simulink library "Byte_Multiplexers_Lib"  (R2023a)
settings: Solver=ode45  StartTime=0.0  StopTime=10.0  RelTol=1e-3  EnableMultiTasking=on
settings Model: Creator=uzivatel  LastModifiedBy=Jozko Mrkvicka
settings SolverCC: AlgebraicLoopSolver=TrustRegion
settings DataIOCC: LimitDataPoints=on  SaveFormat=Array  ReturnWorkspaceOutputs=off
settings OptimizationCC: LifeSpan=inf
settings DebuggingCC: UnderspecifiedInitializationDetection=Classic  MergeDetectMultiDrivingBlocksExec=none  SolverPrmCheckMsg=warning  UnconnectedInputMsg=warning  UnconnectedOutputMsg=warning  UnconnectedLineMsg=warning  StateNameClashWarn=warning  SFUnexpectedBacktrackingDiag=warning  SFNoUnconditionalDefaultTransitionDiag=warning  ArithmeticOperatorsInVariantConditions=warning
settings HardwareCC: ProdBitPerPointer=32  ProdBitPerSizeT=32  ProdBitPerPtrDiffT=32  ProdLargestAtomicFloat=None  ProdIntDivRoundTo=Undefined  ProdEndianess=Unspecified  ProdWordSize=32  ProdHWDeviceType=32-bit Generic
settings ModelReferenceCC: EnableRefExpFcnMdlSchedulingChecks=on  PropagateSignalLabelsOutOfModel=off
settings SFSimCC: SimUseLocalCustomCode=off  CustomCodeUndefinedFunction=UseInterfaceOnly
settings RTWCC: RTWUseLocalCustomCode=off
settings CodeAppCC: StateflowObjectComments=on
settings GRTTargetCC: TargetLangStandard=C89/C90 (ANSI)
settings ConfigComp: CovMetricSettings=dw  CovSaveCumulativeToWorkspaceVar=on  CovSaveSingleToWorkspaceVar=on  CovExternalEMLEnable=off

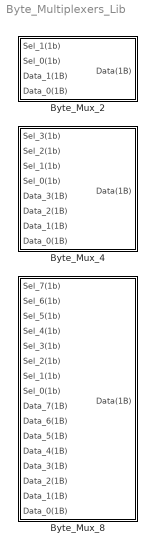
== system Byte_Multiplexers_Lib ==
  Byte_Mux_2 : Subsystem
  Byte_Mux_4 : Subsystem
  Byte_Mux_8 : Subsystem

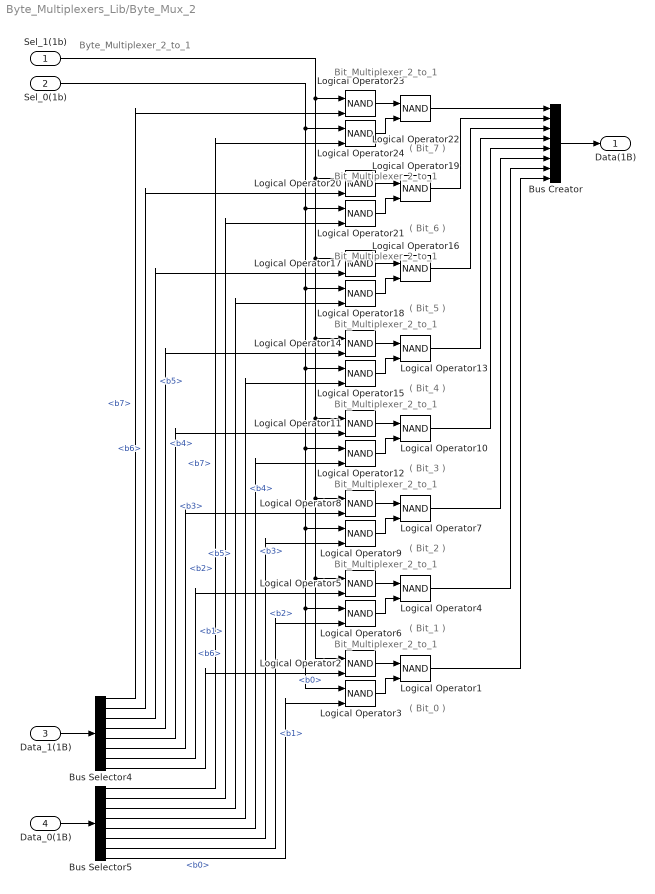
== system Byte_Multiplexers_Lib/Byte_Mux_2 ==
  note: ( Bit_0 )
  note: Bit_Multiplexer_2_to_1
  note: ( Bit_1 )
  note: Bit_Multiplexer_2_to_1
  note: ( Bit_2 )
  note: Bit_Multiplexer_2_to_1
  note: ( Bit_3 )
  note: Bit_Multiplexer_2_to_1
  note: ( Bit_4 )
  note: Bit_Multiplexer_2_to_1
  note: ( Bit_5 )
  note: Bit_Multiplexer_2_to_1
  note: ( Bit_6 )
  note: Bit_Multiplexer_2_to_1
  note: ( Bit_7 )
  note: Bit_Multiplexer_2_to_1
  note: Byte_Multiplexer_2_to_1
  Sel_1(1b) : Inport
  Sel_0(1b) : Inport  Port=2
  Data_1(1B) : Inport  Port=3
  Data_0(1B) : Inport  Port=4
  Bus Creator : BusCreator  Inputs=8
  Bus Selector4 : BusSelector  OutputSignals=b7,b6,b5,b4,b3,b2,b1,b0
  Bus Selector5 : BusSelector  OutputSignals=b7,b6,b5,b4,b3,b2,b1,b0
  Logical Operator{1..24} (24 alike) : Logic  Operator=NAND  IconShape=distinctive  AllPortsSameDT=off  OutDataTypeStr=boolean
  Data(1B) : Outport
  wires:
  Bus Creator/1 -> Data(1B)/1
  Bus Selector5/8 -> Logical Operator3/2  "<b0>"
  Bus Selector4/8 -> Logical Operator2/2  "<b0>"
  Bus Selector5/7 -> Logical Operator6/2  "<b1>"
  Bus Selector4/7 -> Logical Operator5/2  "<b1>"
  Bus Selector5/6 -> Logical Operator9/2  "<b2>"
  Bus Selector4/6 -> Logical Operator8/2  "<b2>"
  Bus Selector5/5 -> Logical Operator12/2  "<b3>"
  Bus Selector4/5 -> Logical Operator11/2  "<b3>"
  Bus Selector5/4 -> Logical Operator15/2  "<b4>"
  Bus Selector4/4 -> Logical Operator14/2  "<b4>"
  Bus Selector5/3 -> Logical Operator18/2  "<b5>"
  Bus Selector4/3 -> Logical Operator17/2  "<b5>"
  Bus Selector5/2 -> Logical Operator21/2  "<b6>"
  Bus Selector4/2 -> Logical Operator20/2  "<b6>"
  Bus Selector5/1 -> Logical Operator24/2  "<b7>"
  Bus Selector4/1 -> Logical Operator23/2  "<b7>"
  Sel_0(1b)/1 -> Logical Operator24/1, Logical Operator21/1, Logical Operator18/1, Logical Operator15/1, Logical Operator12/1, Logical Operator9/1, Logical Operator3/1, Logical Operator6/1
  Logical Operator19/1 -> Bus Creator/2
  Logical Operator13/1 -> Bus Creator/4
  Logical Operator7/1 -> Bus Creator/6
  Logical Operator1/1 -> Bus Creator/8
  Logical Operator4/1 -> Bus Creator/7
  Logical Operator10/1 -> Bus Creator/5
  Logical Operator16/1 -> Bus Creator/3
  Logical Operator22/1 -> Bus Creator/1
  Data_0(1B)/1 -> Bus Selector5/1
  Data_1(1B)/1 -> Bus Selector4/1
  Logical Operator3/1 -> Logical Operator1/2
  Logical Operator2/1 -> Logical Operator1/1
  Logical Operator6/1 -> Logical Operator4/2
  Logical Operator5/1 -> Logical Operator4/1
  Logical Operator9/1 -> Logical Operator7/2
  Logical Operator8/1 -> Logical Operator7/1
  Logical Operator12/1 -> Logical Operator10/2
  Logical Operator11/1 -> Logical Operator10/1
  Logical Operator15/1 -> Logical Operator13/2
  Logical Operator14/1 -> Logical Operator13/1
  Logical Operator18/1 -> Logical Operator16/2
  Logical Operator17/1 -> Logical Operator16/1
  Logical Operator21/1 -> Logical Operator19/2
  Logical Operator20/1 -> Logical Operator19/1
  Logical Operator24/1 -> Logical Operator22/2
  Logical Operator23/1 -> Logical Operator22/1
  Sel_1(1b)/1 -> Logical Operator23/1, Logical Operator20/1, Logical Operator11/1, Logical Operator8/1, Logical Operator5/1, Logical Operator2/1, Logical Operator14/1, Logical Operator17/1

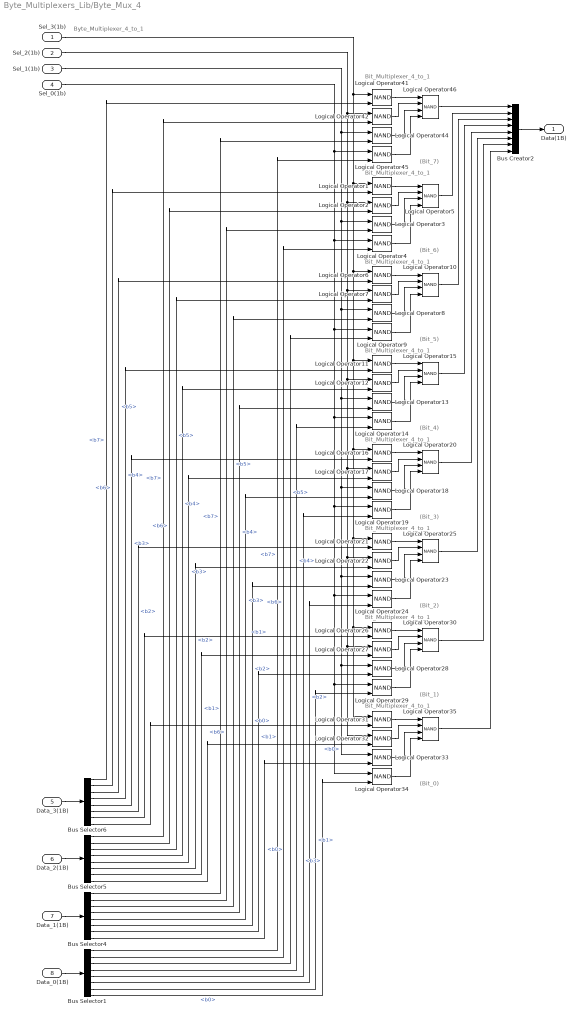
== system Byte_Multiplexers_Lib/Byte_Mux_4 ==
  note: (Bit_7)
  note: Bit_Multiplexer_4_to_1
  note: Bit_Multiplexer_4_to_1
  note: (Bit_6)
  note: Bit_Multiplexer_4_to_1
  note: (Bit_5)
  note: Bit_Multiplexer_4_to_1
  note: (Bit_4)
  note: Bit_Multiplexer_4_to_1
  note: (Bit_3)
  note: Bit_Multiplexer_4_to_1
  note: (Bit_2)
  note: Bit_Multiplexer_4_to_1
  note: (Bit_1)
  note: Bit_Multiplexer_4_to_1
  note: (Bit_0)
  note: Byte_Multiplexer_4_to_1
  Sel_3(1b) : Inport
  Sel_2(1b) : Inport  Port=2
  Sel_1(1b) : Inport  Port=3
  Sel_0(1b) : Inport  Port=4
  Data_3(1B) : Inport  Port=5
  Data_2(1B) : Inport  Port=6
  Data_1(1B) : Inport  Port=7
  Data_0(1B) : Inport  Port=8
  Bus Creator2 : BusCreator  Inputs=8
  Bus Selector{1,4..6} (4 alike) : BusSelector  OutputSignals=b7,b6,b5,b4,b3,b2,b1,b0
  Logical Operator{1..4,6..9,11..14,16..19,21..24,26..29,31..34,41..42,44..45} (32 alike) : Logic  Operator=NAND  IconShape=distinctive  AllPortsSameDT=off  OutDataTypeStr=boolean
  Logical Operator{5,10,15,20,25,30,35,46} (8 alike) : Logic  Operator=NAND  Inputs=4  IconShape=distinctive  OutDataTypeStr=boolean
  Data(1B) : Outport
  wires:
  Bus Creator2/1 -> Data(1B)/1
  Bus Selector1/8 -> Logical Operator34/2  "<b0>"
  Bus Selector4/8 -> Logical Operator33/2  "<b0>"
  Bus Selector5/8 -> Logical Operator32/2  "<b0>"
  Bus Selector6/8 -> Logical Operator31/2  "<b0>"
  Bus Selector1/7 -> Logical Operator29/2  "<b1>"
  Bus Selector4/7 -> Logical Operator28/2  "<b1>"
  Bus Selector5/7 -> Logical Operator27/2  "<b1>"
  Bus Selector6/7 -> Logical Operator26/2  "<b1>"
  Bus Selector1/6 -> Logical Operator24/2  "<b2>"
  Bus Selector4/6 -> Logical Operator23/2  "<b2>"
  Bus Selector5/6 -> Logical Operator22/2  "<b2>"
  Bus Selector6/6 -> Logical Operator21/2  "<b2>"
  Bus Selector1/5 -> Logical Operator19/2  "<b3>"
  Bus Selector4/5 -> Logical Operator18/2  "<b3>"
  Bus Selector5/5 -> Logical Operator17/2  "<b3>"
  Bus Selector6/5 -> Logical Operator16/2  "<b3>"
  Bus Selector1/4 -> Logical Operator14/2  "<b4>"
  Bus Selector4/4 -> Logical Operator13/2  "<b4>"
  Bus Selector5/4 -> Logical Operator12/2  "<b4>"
  Bus Selector6/4 -> Logical Operator11/2  "<b4>"
  Bus Selector1/3 -> Logical Operator9/2  "<b5>"
  Bus Selector4/3 -> Logical Operator8/2  "<b5>"
  Bus Selector5/3 -> Logical Operator7/2  "<b5>"
  Bus Selector6/3 -> Logical Operator6/2  "<b5>"
  Bus Selector1/2 -> Logical Operator4/2  "<b6>"
  Bus Selector4/2 -> Logical Operator3/2  "<b6>"
  Bus Selector5/2 -> Logical Operator2/2  "<b6>"
  Bus Selector6/2 -> Logical Operator1/2  "<b6>"
  Bus Selector1/1 -> Logical Operator45/2  "<b7>"
  Bus Selector4/1 -> Logical Operator44/2  "<b7>"
  Bus Selector5/1 -> Logical Operator42/2  "<b7>"
  Bus Selector6/1 -> Logical Operator41/2  "<b7>"
  Sel_3(1b)/1 -> Logical Operator41/1, Logical Operator1/1, Logical Operator6/1, Logical Operator11/1, Logical Operator21/1, Logical Operator26/1, Logical Operator31/1, Logical Operator16/1
  Sel_2(1b)/1 -> Logical Operator12/1, Logical Operator22/1, Logical Operator27/1, Logical Operator32/1, Logical Operator17/1, Logical Operator7/1, Logical Operator2/1, Logical Operator42/1
  Sel_0(1b)/1 -> Logical Operator34/1, Logical Operator29/1, Logical Operator24/1, Logical Operator19/1, Logical Operator14/1, Logical Operator9/1, Logical Operator4/1, Logical Operator45/1
  Logical Operator5/1 -> Bus Creator2/2
  Logical Operator15/1 -> Bus Creator2/4
  Logical Operator25/1 -> Bus Creator2/6
  Logical Operator35/1 -> Bus Creator2/8
  Sel_1(1b)/1 -> Logical Operator28/1, Logical Operator33/1, Logical Operator23/1, Logical Operator18/1, Logical Operator13/1, Logical Operator8/1, Logical Operator3/1, Logical Operator44/1
  Logical Operator30/1 -> Bus Creator2/7
  Logical Operator20/1 -> Bus Creator2/5
  Logical Operator10/1 -> Bus Creator2/3
  Logical Operator46/1 -> Bus Creator2/1
  Data_0(1B)/1 -> Bus Selector1/1
  Data_1(1B)/1 -> Bus Selector4/1
  Data_2(1B)/1 -> Bus Selector5/1
  Data_3(1B)/1 -> Bus Selector6/1
  Logical Operator45/1 -> Logical Operator46/4
  Logical Operator41/1 -> Logical Operator46/1
  Logical Operator44/1 -> Logical Operator46/3
  Logical Operator42/1 -> Logical Operator46/2
  Logical Operator2/1 -> Logical Operator5/2
  Logical Operator4/1 -> Logical Operator5/4
  Logical Operator3/1 -> Logical Operator5/3
  Logical Operator1/1 -> Logical Operator5/1
  Logical Operator7/1 -> Logical Operator10/2
  Logical Operator9/1 -> Logical Operator10/4
  Logical Operator8/1 -> Logical Operator10/3
  Logical Operator6/1 -> Logical Operator10/1
  Logical Operator12/1 -> Logical Operator15/2
  Logical Operator14/1 -> Logical Operator15/4
  Logical Operator13/1 -> Logical Operator15/3
  Logical Operator11/1 -> Logical Operator15/1
  Logical Operator17/1 -> Logical Operator20/2
  Logical Operator19/1 -> Logical Operator20/4
  Logical Operator18/1 -> Logical Operator20/3
  Logical Operator16/1 -> Logical Operator20/1
  Logical Operator22/1 -> Logical Operator25/2
  Logical Operator24/1 -> Logical Operator25/4
  Logical Operator23/1 -> Logical Operator25/3
  Logical Operator21/1 -> Logical Operator25/1
  Logical Operator27/1 -> Logical Operator30/2
  Logical Operator29/1 -> Logical Operator30/4
  Logical Operator28/1 -> Logical Operator30/3
  Logical Operator26/1 -> Logical Operator30/1
  Logical Operator32/1 -> Logical Operator35/2
  Logical Operator34/1 -> Logical Operator35/4
  Logical Operator33/1 -> Logical Operator35/3
  Logical Operator31/1 -> Logical Operator35/1

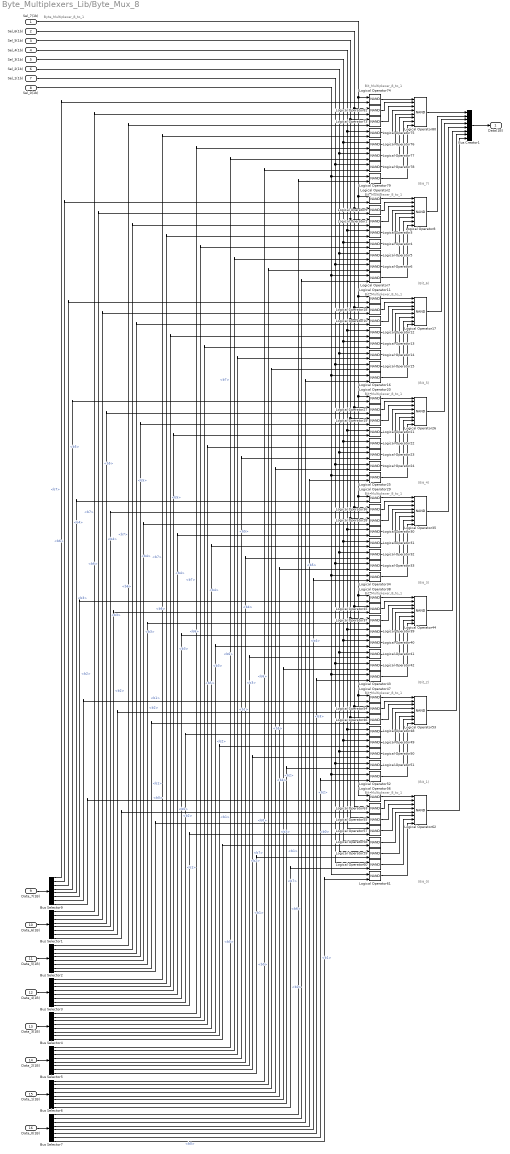
== system Byte_Multiplexers_Lib/Byte_Mux_8 ==
  note: Bit_Multiplexer_8_to_1
  note: (Bit_7)
  note: Bit_Multiplexer_8_to_1
  note: (Bit_6)
  note: Bit_Multiplexer_8_to_1
  note: (Bit_5)
  note: Bit_Multiplexer_8_to_1
  note: (Bit_4)
  note: Bit_Multiplexer_8_to_1
  note: (Bit_3)
  note: Bit_Multiplexer_8_to_1
  note: (Bit_2)
  note: Bit_Multiplexer_8_to_1
  note: (Bit_1)
  note: Bit_Multiplexer_8_to_1
  note: (Bit_0)
  note: Byte_Multiplexer_8_to_1
  Sel_7(1b) : Inport
  Sel_6(1b) : Inport  Port=2
  Sel_5(1b) : Inport  Port=3
  Sel_4(1b) : Inport  Port=4
  Sel_3(1b) : Inport  Port=5
  Sel_2(1b) : Inport  Port=6
  Sel_1(1b) : Inport  Port=7
  Sel_0(1b) : Inport  Port=8
  Data_7(1B) : Inport  Port=9
  Data_6(1B) : Inport  Port=10
  Data_5(1B) : Inport  Port=11
  Data_4(1B) : Inport  Port=12
  Data_3(1B) : Inport  Port=13
  Data_2(1B) : Inport  Port=14
  Data_1(1B) : Inport  Port=15
  Data_0(1B) : Inport  Port=16
  Bus Creator1 : BusCreator  Inputs=8
  Bus Selector{1..7,9} (8 alike) : BusSelector  OutputSignals=b7,b6,b5,b4,b3,b2,b1,b0
  Logical Operator{1..7,9..16,18..25,27..34,36..43,45..52,54..61,63,73..79,81} (64 alike) : Logic  Operator=NAND  IconShape=distinctive  AllPortsSameDT=off  OutDataTypeStr=boolean
  Logical Operator{8,17,26,35,44,53,62,80} (8 alike) : Logic  Operator=NAND  Inputs=8  IconShape=distinctive  OutDataTypeStr=boolean
  Data(1B) : Outport
  wires:
  Bus Creator1/1 -> Data(1B)/1
  Bus Selector7/8 -> Logical Operator61/2  "<b0>"
  Bus Selector6/8 -> Logical Operator60/2  "<b0>"
  Bus Selector5/8 -> Logical Operator59/2  "<b0>"
  Bus Selector4/8 -> Logical Operator58/2  "<b0>"
  Bus Selector3/8 -> Logical Operator57/2  "<b0>"
  Bus Selector2/8 -> Logical Operator55/2  "<b0>"
  Bus Selector1/8 -> Logical Operator63/2  "<b0>"
  Bus Selector9/8 -> Logical Operator56/2  "<b0>"
  Bus Selector7/7 -> Logical Operator52/2  "<b1>"
  Bus Selector6/7 -> Logical Operator51/2  "<b1>"
  Bus Selector5/7 -> Logical Operator50/2  "<b1>"
  Bus Selector4/7 -> Logical Operator49/2  "<b1>"
  Bus Selector3/7 -> Logical Operator48/2  "<b1>"
  Bus Selector2/7 -> Logical Operator46/2  "<b1>"
  Bus Selector1/7 -> Logical Operator54/2  "<b1>"
  Bus Selector9/7 -> Logical Operator47/2  "<b1>"
  Bus Selector7/6 -> Logical Operator43/2  "<b2>"
  Bus Selector6/6 -> Logical Operator42/2  "<b2>"
  Bus Selector5/6 -> Logical Operator41/2  "<b2>"
  Bus Selector4/6 -> Logical Operator40/2  "<b2>"
  Bus Selector3/6 -> Logical Operator39/2  "<b2>"
  Bus Selector2/6 -> Logical Operator37/2  "<b2>"
  Bus Selector1/6 -> Logical Operator45/2  "<b2>"
  Bus Selector9/6 -> Logical Operator38/2  "<b2>"
  Bus Selector7/5 -> Logical Operator34/2  "<b3>"
  Bus Selector6/5 -> Logical Operator33/2  "<b3>"
  Bus Selector5/5 -> Logical Operator32/2  "<b3>"
  Bus Selector4/5 -> Logical Operator31/2  "<b3>"
  Bus Selector3/5 -> Logical Operator30/2  "<b3>"
  Bus Selector2/5 -> Logical Operator28/2  "<b3>"
  Bus Selector1/5 -> Logical Operator36/2  "<b3>"
  Bus Selector9/5 -> Logical Operator29/2  "<b3>"
  Bus Selector7/4 -> Logical Operator25/2  "<b4>"
  Bus Selector6/4 -> Logical Operator24/2  "<b4>"
  Bus Selector5/4 -> Logical Operator23/2  "<b4>"
  Bus Selector4/4 -> Logical Operator22/2  "<b4>"
  Bus Selector3/4 -> Logical Operator21/2  "<b4>"
  Bus Selector2/4 -> Logical Operator19/2  "<b4>"
  Bus Selector1/4 -> Logical Operator27/2  "<b4>"
  Bus Selector9/4 -> Logical Operator20/2  "<b4>"
  Bus Selector7/3 -> Logical Operator16/2  "<b5>"
  Bus Selector6/3 -> Logical Operator15/2  "<b5>"
  Bus Selector5/3 -> Logical Operator14/2  "<b5>"
  Bus Selector4/3 -> Logical Operator13/2  "<b5>"
  Bus Selector3/3 -> Logical Operator12/2  "<b5>"
  Bus Selector2/3 -> Logical Operator10/2  "<b5>"
  Bus Selector1/3 -> Logical Operator18/2  "<b5>"
  Bus Selector9/3 -> Logical Operator11/2  "<b5>"
  Bus Selector7/2 -> Logical Operator7/2  "<b6>"
  Bus Selector6/2 -> Logical Operator6/2  "<b6>"
  Bus Selector5/2 -> Logical Operator5/2  "<b6>"
  Bus Selector4/2 -> Logical Operator4/2  "<b6>"
  Bus Selector3/2 -> Logical Operator3/2  "<b6>"
  Bus Selector2/2 -> Logical Operator1/2  "<b6>"
  Bus Selector1/2 -> Logical Operator9/2  "<b6>"
  Bus Selector9/2 -> Logical Operator2/2  "<b6>"
  Bus Selector7/1 -> Logical Operator79/2  "<b7>"
  Bus Selector6/1 -> Logical Operator78/2  "<b7>"
  Bus Selector5/1 -> Logical Operator77/2  "<b7>"
  Bus Selector4/1 -> Logical Operator76/2  "<b7>"
  Bus Selector3/1 -> Logical Operator75/2  "<b7>"
  Bus Selector2/1 -> Logical Operator73/2  "<b7>"
  Bus Selector1/1 -> Logical Operator81/2  "<b7>"
  Bus Selector9/1 -> Logical Operator74/2  "<b7>"
  Sel_7(1b)/1 -> Logical Operator56/1, Logical Operator47/1, Logical Operator38/1, Logical Operator29/1, Logical Operator20/1, Logical Operator11/1, Logical Operator2/1, Logical Operator74/1
  Sel_6(1b)/1 -> Logical Operator63/1, Logical Operator54/1, Logical Operator45/1, Logical Operator36/1, Logical Operator27/1, Logical Operator18/1, Logical Operator9/1, Logical Operator81/1
  Sel_4(1b)/1 -> Logical Operator57/1, Logical Operator48/1, Logical Operator39/1, Logical Operator30/1, Logical Operator21/1, Logical Operator12/1, Logical Operator3/1, Logical Operator75/1
  Sel_3(1b)/1 -> Logical Operator58/1, Logical Operator49/1, Logical Operator40/1, Logical Operator31/1, Logical Operator22/1, Logical Operator13/1, Logical Operator4/1, Logical Operator76/1
  Sel_2(1b)/1 -> Logical Operator5/1, Logical Operator14/1, Logical Operator23/1, Logical Operator59/1, Logical Operator50/1, Logical Operator41/1, Logical Operator32/1, Logical Operator77/1
  Sel_0(1b)/1 -> Logical Operator79/1, Logical Operator7/1, Logical Operator25/1, Logical Operator34/1, Logical Operator43/1, Logical Operator61/1, Logical Operator52/1, Logical Operator16/1
  Logical Operator8/1 -> Bus Creator1/2
  Logical Operator26/1 -> Bus Creator1/4
  Logical Operator44/1 -> Bus Creator1/6
  Logical Operator62/1 -> Bus Creator1/8
  Sel_1(1b)/1 -> Logical Operator60/1, Logical Operator51/1, Logical Operator42/1, Logical Operator33/1, Logical Operator24/1, Logical Operator15/1, Logical Operator6/1, Logical Operator78/1
  Sel_5(1b)/1 -> Logical Operator55/1, Logical Operator46/1, Logical Operator37/1, Logical Operator28/1, Logical Operator19/1, Logical Operator10/1, Logical Operator1/1, Logical Operator73/1
  Logical Operator53/1 -> Bus Creator1/7
  Logical Operator35/1 -> Bus Creator1/5
  Logical Operator17/1 -> Bus Creator1/3
  Logical Operator80/1 -> Bus Creator1/1
  Data_0(1B)/1 -> Bus Selector7/1
  Logical Operator73/1 -> Logical Operator80/3
  Logical Operator74/1 -> Logical Operator80/1
  Logical Operator78/1 -> Logical Operator80/7
  Logical Operator76/1 -> Logical Operator80/5
  Logical Operator81/1 -> Logical Operator80/2
  Logical Operator75/1 -> Logical Operator80/4
  Logical Operator77/1 -> Logical Operator80/6
  Logical Operator79/1 -> Logical Operator80/8
  Logical Operator1/1 -> Logical Operator8/3
  Logical Operator2/1 -> Logical Operator8/1
  Logical Operator6/1 -> Logical Operator8/7
  Logical Operator4/1 -> Logical Operator8/5
  Logical Operator9/1 -> Logical Operator8/2
  Logical Operator3/1 -> Logical Operator8/4
  Logical Operator5/1 -> Logical Operator8/6
  Logical Operator7/1 -> Logical Operator8/8
  Logical Operator10/1 -> Logical Operator17/3
  Logical Operator11/1 -> Logical Operator17/1
  Logical Operator15/1 -> Logical Operator17/7
  Logical Operator13/1 -> Logical Operator17/5
  Logical Operator18/1 -> Logical Operator17/2
  Logical Operator12/1 -> Logical Operator17/4
  Logical Operator14/1 -> Logical Operator17/6
  Logical Operator16/1 -> Logical Operator17/8
  Logical Operator19/1 -> Logical Operator26/3
  Logical Operator20/1 -> Logical Operator26/1
  Logical Operator24/1 -> Logical Operator26/7
  Logical Operator22/1 -> Logical Operator26/5
  Logical Operator27/1 -> Logical Operator26/2
  Logical Operator21/1 -> Logical Operator26/4
  Logical Operator23/1 -> Logical Operator26/6
  Logical Operator25/1 -> Logical Operator26/8
  Logical Operator28/1 -> Logical Operator35/3
  Logical Operator29/1 -> Logical Operator35/1
  Logical Operator33/1 -> Logical Operator35/7
  Logical Operator31/1 -> Logical Operator35/5
  Logical Operator36/1 -> Logical Operator35/2
  Logical Operator30/1 -> Logical Operator35/4
  Logical Operator32/1 -> Logical Operator35/6
  Logical Operator34/1 -> Logical Operator35/8
  Logical Operator37/1 -> Logical Operator44/3
  Logical Operator38/1 -> Logical Operator44/1
  Logical Operator42/1 -> Logical Operator44/7
  Logical Operator40/1 -> Logical Operator44/5
  Logical Operator45/1 -> Logical Operator44/2
  Logical Operator39/1 -> Logical Operator44/4
  Logical Operator41/1 -> Logical Operator44/6
  Logical Operator43/1 -> Logical Operator44/8
  Logical Operator46/1 -> Logical Operator53/3
  Logical Operator47/1 -> Logical Operator53/1
  Logical Operator51/1 -> Logical Operator53/7
  Logical Operator49/1 -> Logical Operator53/5
  Logical Operator54/1 -> Logical Operator53/2
  Logical Operator48/1 -> Logical Operator53/4
  Logical Operator50/1 -> Logical Operator53/6
  Logical Operator52/1 -> Logical Operator53/8
  Logical Operator55/1 -> Logical Operator62/3
  Logical Operator56/1 -> Logical Operator62/1
  Logical Operator60/1 -> Logical Operator62/7
  Logical Operator58/1 -> Logical Operator62/5
  Logical Operator63/1 -> Logical Operator62/2
  Logical Operator57/1 -> Logical Operator62/4
  Logical Operator59/1 -> Logical Operator62/6
  Logical Operator61/1 -> Logical Operator62/8
  Data_6(1B)/1 -> Bus Selector1/1
  Data_5(1B)/1 -> Bus Selector2/1
  Data_4(1B)/1 -> Bus Selector3/1
  Data_3(1B)/1 -> Bus Selector4/1
  Data_2(1B)/1 -> Bus Selector5/1
  Data_1(1B)/1 -> Bus Selector6/1
  Data_7(1B)/1 -> Bus Selector9/1
